simulink model "MSE483_LinearSimulink"  (R2020b)
settings: Solver=ode45  StartTime=0.0  StopTime=10  MaxStep=1e-5  RelTol=1e-3
InitFcn:
  | g = 9.81; %gravity
  | m = 0.03; % wheel weight
  | R = 0.04; % wheel radius
  | J_w = (m*(R^2))/2; % wheel inertia moment
  | M = 0.6; % body weight
  | W = 0.14; % body width
  | D = 0.04; % body depth
  | H = 0.144; % body height
  | L = H/2; % distance to the CoM from wheel axel
  | J_psi = (M*(L^2))/3; % body pitch inertia moment
  | J_phi = (M*(W^2 + D^2))/12; % body yaw inertia moment
  | J_m = 1e-5; % DC motor inertia moment
  | R_m = 6.69; % DC motor resistance
  | K_b = 0.468; % DC motor back EMF constant
  | K_t = 0.317; % DC motor torque constant
  | n = 1; % gear ratio
  | f_m = 0.0022; % friction coefficient between body and motor
  | f_w = 0; % friction coefficient between wheel and floor
  | 
  | a = (n*K_t)/R_m ;
  | b = ((n*K_t*K_b)/R_m) + f_m;
  | 
  | A=[0,  0,           1,          0;
  |     0,  0,           0,          1;
  |     0, -409.7184,  -104.6299,   104.6299;
  |     0,  268.6273,    54.5833,   -54.5833]
  | B = [0;0;101.6952;-53.0523]
  | C=[1 0 0 0]
  | D=[0]
  | x0=[0;90*pi/180;0;0]
  | K=[-318.517516293979	-839.316963783976	-66.2263834004483	-127.491021126397]
  | KI = 890.808276084874
  | Ob= [ 400.0000   ,      0   , 1.0000  , 0;
  |          0 , 400.0000   ,      0  ,  1.0000;
  |          0, -409.718, 295.3701 , 104.6299;
  |          0,  268.6273 ,  54.5833 , 345.4167]
settings Model: Creator=mkupp  LastModifiedBy=mkupp
settings SolverCC: AlgebraicLoopSolver=LineSearch

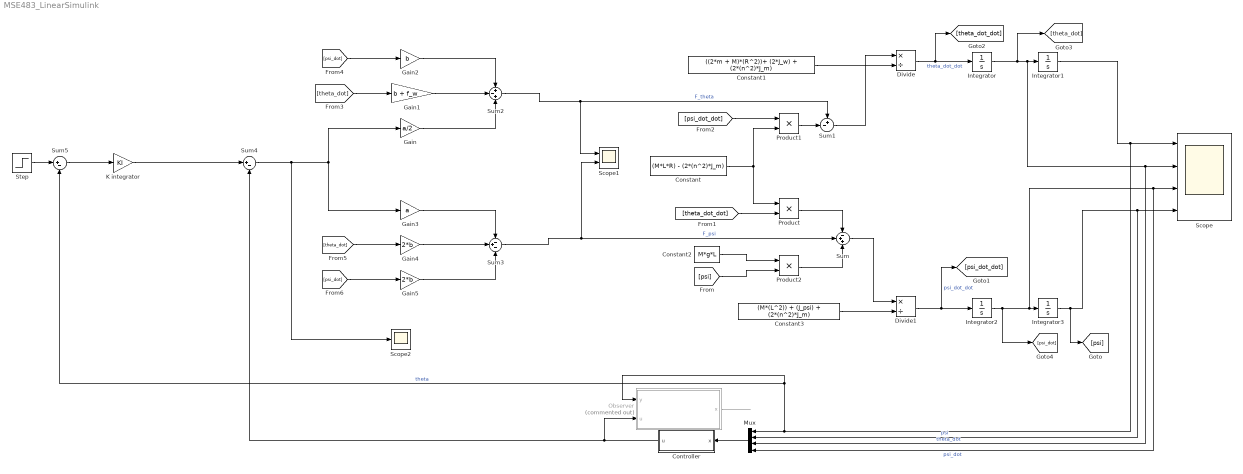
== system MSE483_LinearSimulink ==
  Constant : Constant  Value=(M*L*R) - (2*(n^2)*J_m)
  Constant1 : Constant  Value=((2*m + M)*(R^2))+ (2*J_w) + (2*(n^2)*J_m)
  Constant2 : Constant  Value=M*g*L
  Constant3 : Constant  Value=(M*(L^2)) + (J_psi) + (2*(n^2)*J_m)
  Controller : Subsystem
  Divide : Product  Inputs=*/
  Divide1 : Product  Inputs=*/
  Gain : Gain  Gain=a/2
  Gain1 : Gain  Gain=b + f_w
  Gain2 : Gain  Gain=b
  Gain3 : Gain  Gain=a
  Gain4 : Gain  Gain=2*b
  Gain5 : Gain  Gain=2*b
  Integrator{,1..3} (4 alike) : Integrator
  K integrator : Gain  InitFcn=|  Gain=KI
      | A=[0,  0,           1,          0;
      |     0,  0,           0,          1;
      |     0, -409.7184,  -104.6299,   104.6299;
      |     0,  268.6273,    54.5833,   -54.5833]
      | B = [0;0;101.6952;-53.0523]
      | C=[1 0 0 0]
      | D=[0]
      | x0=[0;90*pi/180;0;0]
      | K=[-62.8966122663488	-201.905572339641	-14.9133345772124	-27.6218237282572]
      | Ob= [ 400.0000   ,      0   , 1.0000  ,       0;
      |          0 , 400.0000   ,      0  ,  1.0000;
      |          0, -409.718, 295.3701 , 104.6299;
      |          0,  268.6273 ,  54.5833 , 345.4167]
  Mux : Mux
  Observer : Subsystem  Commented=on
  Product : Product
  Product1 : Product
  Product2 : Product
  Scope : Scope  NumInputPorts=4
  Scope1 : Scope  NumInputPorts=2
  Scope2 : Scope
  Step : Step  SampleTime=0
  Sum : Sum  Inputs=-++
  Sum1 : Sum  Inputs=+-|
  Sum2 : Sum  Inputs=+-+
  Sum3 : Sum  Inputs=-+-
  Sum4 : Sum  Inputs=|+-
  Sum5 : Sum  Inputs=|+-
  wires:
  Integrator/1 -> [theta_dot], Mux/3, Scope/2, Integrator1/1  "theta_dot"
  Integrator2/1 -> [psi_dot], Mux/4, Scope/3, Integrator3/1  "psi_dot"
  Integrator3/1 -> [psi], Mux/2, Scope/4  "psi"
  Integrator1/1 -> Observer/1(y), Sum5/2, Mux/1, Scope/1  "theta"
  Constant/1 -> Product/1, Product1/2
  Constant1/1 -> Divide/2
  Product1/1 -> Sum1/2
  Constant2/1 -> Product2/1
  Constant3/1 -> Divide1/2
  [psi] -> Product2/2
  Sum1/1 -> Divide/1
  [theta_dot_dot] -> Product/2
  [psi_dot_dot] -> Product1/1
  Product/1 -> Sum/1
  Product2/1 -> Sum/3
  Sum/1 -> Divide1/1
  [theta_dot] -> Gain1/1
  [psi_dot] -> Gain2/1
  Gain2/1 -> Sum2/1
  Gain1/1 -> Sum2/2
  Gain/1 -> Sum2/3
  Gain3/1 -> Sum3/1
  [psi_dot] -> Gain5/1
  [theta_dot] -> Gain4/1
  Gain4/1 -> Sum3/2
  Gain5/1 -> Sum3/3
  Sum3/1 -> Scope1/2, Sum/2  "F_psi"
  Sum2/1 -> Scope1/1, Sum1/1  "F_theta"
  Divide/1 -> Integrator/1, [theta_dot_dot]  "theta_dot_dot"
  Divide1/1 -> [psi_dot_dot], Integrator2/1  "psi_dot_dot"
  K integrator/1 -> Sum4/1
  Sum4/1 -> Scope2/1, Gain3/1, Gain/1
  Mux/1 -> Controller/1(x)
  Sum5/1 -> K integrator/1
  Step/1 -> Sum5/1
  Controller/1(u) -> Observer/2(u), Sum4/2
  Observer/1(x) -> ?

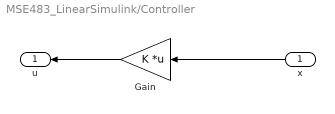
== system MSE483_LinearSimulink/Controller ==
  x : Inport
  Gain : Gain  Gain=K  Multiplication=Matrix(K*u)
  u : Outport
  wires:
  Gain/1 -> u/1
  x/1 -> Gain/1

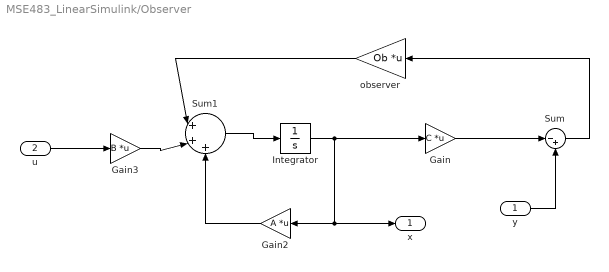
== system MSE483_LinearSimulink/Observer ==
  y : Inport
  u : Inport  Port=2
  Gain : Gain  Gain=C  Multiplication=Matrix(K*u)
  Gain2 : Gain  Gain=A  Multiplication=Matrix(K*u)
  Gain3 : Gain  Gain=B  Multiplication=Matrix(K*u)
  Integrator : Integrator  InitialCondition=x0
  Sum : Sum  Inputs=|-+
  Sum1 : Sum  Inputs=|+++
  observer : Gain  Gain=Ob  Multiplication=Matrix(K*u)
  x : Outport
  wires:
  u/1 -> Gain3/1
  Gain/1 -> Sum/1
  Sum1/1 -> Integrator/1
  Integrator/1 -> Gain2/1, x/1, Gain/1
  y/1 -> Sum/2
  Sum/1 -> observer/1
  observer/1 -> Sum1/1
  Gain3/1 -> Sum1/2
  Gain2/1 -> Sum1/3
